simulink model "pattern3x3_training_2023clock"  (R2024a)
settings: Solver=FixedStepAuto  StartTime=0.0  StopTime=2  FixedStep=0.000005  RelTol=1e-3
model workspace (MAT data in the model file):
  part1_v1 = 1
values from neighbouring files (symbols this model uses):
  full_pattern = load('Pattern4_250.CSV')    [model_setup4.m]
  max_weight2 = 255    [model_setup4.m]
  min_weight2 = 150    [model_setup4.m]
  Th_minus_count2 = 10    [model_setup4.m]    (also in model_setup_test.m = 5)
  Th_plus_count2 = 20    [model_setup4.m]    (also in model_setup_test.m)
libraries: simulink x1
(part 6 of 9)

== system pattern3x3_training_2023clock/Synapse11/Clock2 ==
  clock : Inport
  "Reset " : Inport  Port=2
  Memory2 : Memory
  NOT1 : Logic  Operator=NOT  IconShape=distinctive  AllPortsSameDT=off  OutDataTypeStr=boolean
  Product1 : Product
  Triggered Subsystem1 : Subsystem  TreatAsAtomicUnit=on
  T : Outport  VectorParamsAs1DForOutWhenUnconnected=off
  wires:
  Memory2/1 -> Triggered Subsystem1/1(In1)
  Product1/1 -> T/1, Memory2/1
  "Reset "/1 -> NOT1/1
  Triggered Subsystem1/1(Out1) -> Product1/1
  NOT1/1 -> Product1/2
  clock/1 -> Triggered Subsystem1/Trigger

== system pattern3x3_training_2023clock/Synapse11/Clock3 ==
  clock : Inport
  "Reset " : Inport  Port=2
  Memory2 : Memory
  NOT1 : Logic  Operator=NOT  IconShape=distinctive  AllPortsSameDT=off  OutDataTypeStr=boolean
  Product1 : Product
  Triggered Subsystem1 : Subsystem  TreatAsAtomicUnit=on
  T : Outport  VectorParamsAs1DForOutWhenUnconnected=off
  wires:
  Memory2/1 -> Triggered Subsystem1/1(In1)
  Product1/1 -> T/1, Memory2/1
  "Reset "/1 -> NOT1/1
  Triggered Subsystem1/1(Out1) -> Product1/1
  NOT1/1 -> Product1/2
  clock/1 -> Triggered Subsystem1/Trigger

== system pattern3x3_training_2023clock/Synapse11/Subsystem ==
  delta_weight : Inport
  before_weight : Inport  Port=2
  Trigger : TriggerPort  VariantControl=(inherit)  PortDimensions=1
  Sum : Sum  Inputs=|++
  weight : Outport
  wires:
  delta_weight/1 -> Sum/1
  Sum/1 -> weight/1
  before_weight/1 -> Sum/2

== system pattern3x3_training_2023clock/Synapse12/Clock1 ==
  clock : Inport
  "Reset " : Inport  Port=2
  Memory2 : Memory
  NOT1 : Logic  Operator=NOT  IconShape=distinctive  AllPortsSameDT=off  OutDataTypeStr=boolean
  Product1 : Product
  Triggered Subsystem1 : Subsystem  TreatAsAtomicUnit=on
  T : Outport  VectorParamsAs1DForOutWhenUnconnected=off
  wires:
  Memory2/1 -> Triggered Subsystem1/1(In1)
  Product1/1 -> T/1, Memory2/1
  "Reset "/1 -> NOT1/1
  Triggered Subsystem1/1(Out1) -> Product1/1
  NOT1/1 -> Product1/2
  clock/1 -> Triggered Subsystem1/Trigger

== system pattern3x3_training_2023clock/Synapse12/Clock2 ==
  clock : Inport
  "Reset " : Inport  Port=2
  Memory2 : Memory
  NOT1 : Logic  Operator=NOT  IconShape=distinctive  AllPortsSameDT=off  OutDataTypeStr=boolean
  Product1 : Product
  Triggered Subsystem1 : Subsystem  TreatAsAtomicUnit=on
  T : Outport  VectorParamsAs1DForOutWhenUnconnected=off
  wires:
  Memory2/1 -> Triggered Subsystem1/1(In1)
  Product1/1 -> T/1, Memory2/1
  "Reset "/1 -> NOT1/1
  Triggered Subsystem1/1(Out1) -> Product1/1
  NOT1/1 -> Product1/2
  clock/1 -> Triggered Subsystem1/Trigger

== system pattern3x3_training_2023clock/Synapse12/Clock3 ==
  clock : Inport
  "Reset " : Inport  Port=2
  Memory2 : Memory
  NOT1 : Logic  Operator=NOT  IconShape=distinctive  AllPortsSameDT=off  OutDataTypeStr=boolean
  Product1 : Product
  Triggered Subsystem1 : Subsystem  TreatAsAtomicUnit=on
  T : Outport  VectorParamsAs1DForOutWhenUnconnected=off
  wires:
  Memory2/1 -> Triggered Subsystem1/1(In1)
  Product1/1 -> T/1, Memory2/1
  "Reset "/1 -> NOT1/1
  Triggered Subsystem1/1(Out1) -> Product1/1
  NOT1/1 -> Product1/2
  clock/1 -> Triggered Subsystem1/Trigger

== system pattern3x3_training_2023clock/Synapse12/Subsystem ==
  delta_weight : Inport
  before_weight : Inport  Port=2
  Trigger : TriggerPort  VariantControl=(inherit)  PortDimensions=1
  Sum : Sum  Inputs=|++
  weight : Outport
  wires:
  delta_weight/1 -> Sum/1
  Sum/1 -> weight/1
  before_weight/1 -> Sum/2

== system pattern3x3_training_2023clock/Synapse13/Clock1 ==
  clock : Inport
  "Reset " : Inport  Port=2
  Memory2 : Memory
  NOT1 : Logic  Operator=NOT  IconShape=distinctive  AllPortsSameDT=off  OutDataTypeStr=boolean
  Product1 : Product
  Triggered Subsystem1 : Subsystem  TreatAsAtomicUnit=on
  T : Outport  VectorParamsAs1DForOutWhenUnconnected=off
  wires:
  Memory2/1 -> Triggered Subsystem1/1(In1)
  Product1/1 -> T/1, Memory2/1
  "Reset "/1 -> NOT1/1
  Triggered Subsystem1/1(Out1) -> Product1/1
  NOT1/1 -> Product1/2
  clock/1 -> Triggered Subsystem1/Trigger

== system pattern3x3_training_2023clock/Synapse13/Clock2 ==
  clock : Inport
  "Reset " : Inport  Port=2
  Memory2 : Memory
  NOT1 : Logic  Operator=NOT  IconShape=distinctive  AllPortsSameDT=off  OutDataTypeStr=boolean
  Product1 : Product
  Triggered Subsystem1 : Subsystem  TreatAsAtomicUnit=on
  T : Outport  VectorParamsAs1DForOutWhenUnconnected=off
  wires:
  Memory2/1 -> Triggered Subsystem1/1(In1)
  Product1/1 -> T/1, Memory2/1
  "Reset "/1 -> NOT1/1
  Triggered Subsystem1/1(Out1) -> Product1/1
  NOT1/1 -> Product1/2
  clock/1 -> Triggered Subsystem1/Trigger

== system pattern3x3_training_2023clock/Synapse13/Clock3 ==
  clock : Inport
  "Reset " : Inport  Port=2
  Memory2 : Memory
  NOT1 : Logic  Operator=NOT  IconShape=distinctive  AllPortsSameDT=off  OutDataTypeStr=boolean
  Product1 : Product
  Triggered Subsystem1 : Subsystem  TreatAsAtomicUnit=on
  T : Outport  VectorParamsAs1DForOutWhenUnconnected=off
  wires:
  Memory2/1 -> Triggered Subsystem1/1(In1)
  Product1/1 -> T/1, Memory2/1
  "Reset "/1 -> NOT1/1
  Triggered Subsystem1/1(Out1) -> Product1/1
  NOT1/1 -> Product1/2
  clock/1 -> Triggered Subsystem1/Trigger

== system pattern3x3_training_2023clock/Synapse13/Subsystem ==
  delta_weight : Inport
  before_weight : Inport  Port=2
  Trigger : TriggerPort  VariantControl=(inherit)  PortDimensions=1
  Sum : Sum  Inputs=|++
  weight : Outport
  wires:
  delta_weight/1 -> Sum/1
  Sum/1 -> weight/1
  before_weight/1 -> Sum/2

== system pattern3x3_training_2023clock/Synapse14/Clock1 ==
  clock : Inport
  "Reset " : Inport  Port=2
  Memory2 : Memory
  NOT1 : Logic  Operator=NOT  IconShape=distinctive  AllPortsSameDT=off  OutDataTypeStr=boolean
  Product1 : Product
  Triggered Subsystem1 : Subsystem  TreatAsAtomicUnit=on
  T : Outport  VectorParamsAs1DForOutWhenUnconnected=off
  wires:
  Memory2/1 -> Triggered Subsystem1/1(In1)
  Product1/1 -> T/1, Memory2/1
  "Reset "/1 -> NOT1/1
  Triggered Subsystem1/1(Out1) -> Product1/1
  NOT1/1 -> Product1/2
  clock/1 -> Triggered Subsystem1/Trigger

== system pattern3x3_training_2023clock/Synapse14/Clock2 ==
  clock : Inport
  "Reset " : Inport  Port=2
  Memory2 : Memory
  NOT1 : Logic  Operator=NOT  IconShape=distinctive  AllPortsSameDT=off  OutDataTypeStr=boolean
  Product1 : Product
  Triggered Subsystem1 : Subsystem  TreatAsAtomicUnit=on
  T : Outport  VectorParamsAs1DForOutWhenUnconnected=off
  wires:
  Memory2/1 -> Triggered Subsystem1/1(In1)
  Product1/1 -> T/1, Memory2/1
  "Reset "/1 -> NOT1/1
  Triggered Subsystem1/1(Out1) -> Product1/1
  NOT1/1 -> Product1/2
  clock/1 -> Triggered Subsystem1/Trigger

== system pattern3x3_training_2023clock/Synapse14/Clock3 ==
  clock : Inport
  "Reset " : Inport  Port=2
  Memory2 : Memory
  NOT1 : Logic  Operator=NOT  IconShape=distinctive  AllPortsSameDT=off  OutDataTypeStr=boolean
  Product1 : Product
  Triggered Subsystem1 : Subsystem  TreatAsAtomicUnit=on
  T : Outport  VectorParamsAs1DForOutWhenUnconnected=off
  wires:
  Memory2/1 -> Triggered Subsystem1/1(In1)
  Product1/1 -> T/1, Memory2/1
  "Reset "/1 -> NOT1/1
  Triggered Subsystem1/1(Out1) -> Product1/1
  NOT1/1 -> Product1/2
  clock/1 -> Triggered Subsystem1/Trigger

== system pattern3x3_training_2023clock/Synapse14/Subsystem ==
  delta_weight : Inport
  before_weight : Inport  Port=2
  Trigger : TriggerPort  VariantControl=(inherit)  PortDimensions=1
  Sum : Sum  Inputs=|++
  weight : Outport
  wires:
  delta_weight/1 -> Sum/1
  Sum/1 -> weight/1
  before_weight/1 -> Sum/2

== system pattern3x3_training_2023clock/Synapse15/Clock1 ==
  clock : Inport
  "Reset " : Inport  Port=2
  Memory2 : Memory
  NOT1 : Logic  Operator=NOT  IconShape=distinctive  AllPortsSameDT=off  OutDataTypeStr=boolean
  Product1 : Product
  Triggered Subsystem1 : Subsystem  TreatAsAtomicUnit=on
  T : Outport  VectorParamsAs1DForOutWhenUnconnected=off
  wires:
  Memory2/1 -> Triggered Subsystem1/1(In1)
  Product1/1 -> T/1, Memory2/1
  "Reset "/1 -> NOT1/1
  Triggered Subsystem1/1(Out1) -> Product1/1
  NOT1/1 -> Product1/2
  clock/1 -> Triggered Subsystem1/Trigger

== system pattern3x3_training_2023clock/Synapse15/Clock2 ==
  clock : Inport
  "Reset " : Inport  Port=2
  Memory2 : Memory
  NOT1 : Logic  Operator=NOT  IconShape=distinctive  AllPortsSameDT=off  OutDataTypeStr=boolean
  Product1 : Product
  Triggered Subsystem1 : Subsystem  TreatAsAtomicUnit=on
  T : Outport  VectorParamsAs1DForOutWhenUnconnected=off
  wires:
  Memory2/1 -> Triggered Subsystem1/1(In1)
  Product1/1 -> T/1, Memory2/1
  "Reset "/1 -> NOT1/1
  Triggered Subsystem1/1(Out1) -> Product1/1
  NOT1/1 -> Product1/2
  clock/1 -> Triggered Subsystem1/Trigger

== system pattern3x3_training_2023clock/Synapse15/Clock3 ==
  clock : Inport
  "Reset " : Inport  Port=2
  Memory2 : Memory
  NOT1 : Logic  Operator=NOT  IconShape=distinctive  AllPortsSameDT=off  OutDataTypeStr=boolean
  Product1 : Product
  Triggered Subsystem1 : Subsystem  TreatAsAtomicUnit=on
  T : Outport  VectorParamsAs1DForOutWhenUnconnected=off
  wires:
  Memory2/1 -> Triggered Subsystem1/1(In1)
  Product1/1 -> T/1, Memory2/1
  "Reset "/1 -> NOT1/1
  Triggered Subsystem1/1(Out1) -> Product1/1
  NOT1/1 -> Product1/2
  clock/1 -> Triggered Subsystem1/Trigger

== system pattern3x3_training_2023clock/Synapse15/Subsystem ==
  delta_weight : Inport
  before_weight : Inport  Port=2
  Trigger : TriggerPort  VariantControl=(inherit)  PortDimensions=1
  Sum : Sum  Inputs=|++
  weight : Outport
  wires:
  delta_weight/1 -> Sum/1
  Sum/1 -> weight/1
  before_weight/1 -> Sum/2

== system pattern3x3_training_2023clock/Synapse16/Clock1 ==
  clock : Inport
  "Reset " : Inport  Port=2
  Memory2 : Memory
  NOT1 : Logic  Operator=NOT  IconShape=distinctive  AllPortsSameDT=off  OutDataTypeStr=boolean
  Product1 : Product
  Triggered Subsystem1 : Subsystem  TreatAsAtomicUnit=on
  T : Outport  VectorParamsAs1DForOutWhenUnconnected=off
  wires:
  Memory2/1 -> Triggered Subsystem1/1(In1)
  Product1/1 -> T/1, Memory2/1
  "Reset "/1 -> NOT1/1
  Triggered Subsystem1/1(Out1) -> Product1/1
  NOT1/1 -> Product1/2
  clock/1 -> Triggered Subsystem1/Trigger

== system pattern3x3_training_2023clock/Synapse16/Clock2 ==
  clock : Inport
  "Reset " : Inport  Port=2
  Memory2 : Memory
  NOT1 : Logic  Operator=NOT  IconShape=distinctive  AllPortsSameDT=off  OutDataTypeStr=boolean
  Product1 : Product
  Triggered Subsystem1 : Subsystem  TreatAsAtomicUnit=on
  T : Outport  VectorParamsAs1DForOutWhenUnconnected=off
  wires:
  Memory2/1 -> Triggered Subsystem1/1(In1)
  Product1/1 -> T/1, Memory2/1
  "Reset "/1 -> NOT1/1
  Triggered Subsystem1/1(Out1) -> Product1/1
  NOT1/1 -> Product1/2
  clock/1 -> Triggered Subsystem1/Trigger

== system pattern3x3_training_2023clock/Synapse16/Clock3 ==
  clock : Inport
  "Reset " : Inport  Port=2
  Memory2 : Memory
  NOT1 : Logic  Operator=NOT  IconShape=distinctive  AllPortsSameDT=off  OutDataTypeStr=boolean
  Product1 : Product
  Triggered Subsystem1 : Subsystem  TreatAsAtomicUnit=on
  T : Outport  VectorParamsAs1DForOutWhenUnconnected=off
  wires:
  Memory2/1 -> Triggered Subsystem1/1(In1)
  Product1/1 -> T/1, Memory2/1
  "Reset "/1 -> NOT1/1
  Triggered Subsystem1/1(Out1) -> Product1/1
  NOT1/1 -> Product1/2
  clock/1 -> Triggered Subsystem1/Trigger

== system pattern3x3_training_2023clock/Synapse16/Subsystem ==
  delta_weight : Inport
  before_weight : Inport  Port=2
  Trigger : TriggerPort  VariantControl=(inherit)  PortDimensions=1
  Sum : Sum  Inputs=|++
  weight : Outport
  wires:
  delta_weight/1 -> Sum/1
  Sum/1 -> weight/1
  before_weight/1 -> Sum/2

== system pattern3x3_training_2023clock/Synapse17/Clock1 ==
  clock : Inport
  "Reset " : Inport  Port=2
  Memory2 : Memory
  NOT1 : Logic  Operator=NOT  IconShape=distinctive  AllPortsSameDT=off  OutDataTypeStr=boolean
  Product1 : Product
  Triggered Subsystem1 : Subsystem  TreatAsAtomicUnit=on
  T : Outport  VectorParamsAs1DForOutWhenUnconnected=off
  wires:
  Memory2/1 -> Triggered Subsystem1/1(In1)
  Product1/1 -> T/1, Memory2/1
  "Reset "/1 -> NOT1/1
  Triggered Subsystem1/1(Out1) -> Product1/1
  NOT1/1 -> Product1/2
  clock/1 -> Triggered Subsystem1/Trigger

== system pattern3x3_training_2023clock/Synapse17/Clock2 ==
  clock : Inport
  "Reset " : Inport  Port=2
  Memory2 : Memory
  NOT1 : Logic  Operator=NOT  IconShape=distinctive  AllPortsSameDT=off  OutDataTypeStr=boolean
  Product1 : Product
  Triggered Subsystem1 : Subsystem  TreatAsAtomicUnit=on
  T : Outport  VectorParamsAs1DForOutWhenUnconnected=off
  wires:
  Memory2/1 -> Triggered Subsystem1/1(In1)
  Product1/1 -> T/1, Memory2/1
  "Reset "/1 -> NOT1/1
  Triggered Subsystem1/1(Out1) -> Product1/1
  NOT1/1 -> Product1/2
  clock/1 -> Triggered Subsystem1/Trigger

== system pattern3x3_training_2023clock/Synapse17/Clock3 ==
  clock : Inport
  "Reset " : Inport  Port=2
  Memory2 : Memory
  NOT1 : Logic  Operator=NOT  IconShape=distinctive  AllPortsSameDT=off  OutDataTypeStr=boolean
  Product1 : Product
  Triggered Subsystem1 : Subsystem  TreatAsAtomicUnit=on
  T : Outport  VectorParamsAs1DForOutWhenUnconnected=off
  wires:
  Memory2/1 -> Triggered Subsystem1/1(In1)
  Product1/1 -> T/1, Memory2/1
  "Reset "/1 -> NOT1/1
  Triggered Subsystem1/1(Out1) -> Product1/1
  NOT1/1 -> Product1/2
  clock/1 -> Triggered Subsystem1/Trigger

== system pattern3x3_training_2023clock/Synapse17/Subsystem ==
  delta_weight : Inport
  before_weight : Inport  Port=2
  Trigger : TriggerPort  VariantControl=(inherit)  PortDimensions=1
  Sum : Sum  Inputs=|++
  weight : Outport
  wires:
  delta_weight/1 -> Sum/1
  Sum/1 -> weight/1
  before_weight/1 -> Sum/2

== system pattern3x3_training_2023clock/Synapse18/Clock1 ==
  clock : Inport
  "Reset " : Inport  Port=2
  Memory2 : Memory
  NOT1 : Logic  Operator=NOT  IconShape=distinctive  AllPortsSameDT=off  OutDataTypeStr=boolean
  Product1 : Product
  Triggered Subsystem1 : Subsystem  TreatAsAtomicUnit=on
  T : Outport  VectorParamsAs1DForOutWhenUnconnected=off
  wires:
  Memory2/1 -> Triggered Subsystem1/1(In1)
  Product1/1 -> T/1, Memory2/1
  "Reset "/1 -> NOT1/1
  Triggered Subsystem1/1(Out1) -> Product1/1
  NOT1/1 -> Product1/2
  clock/1 -> Triggered Subsystem1/Trigger

== system pattern3x3_training_2023clock/Synapse18/Clock2 ==
  clock : Inport
  "Reset " : Inport  Port=2
  Memory2 : Memory
  NOT1 : Logic  Operator=NOT  IconShape=distinctive  AllPortsSameDT=off  OutDataTypeStr=boolean
  Product1 : Product
  Triggered Subsystem1 : Subsystem  TreatAsAtomicUnit=on
  T : Outport  VectorParamsAs1DForOutWhenUnconnected=off
  wires:
  Memory2/1 -> Triggered Subsystem1/1(In1)
  Product1/1 -> T/1, Memory2/1
  "Reset "/1 -> NOT1/1
  Triggered Subsystem1/1(Out1) -> Product1/1
  NOT1/1 -> Product1/2
  clock/1 -> Triggered Subsystem1/Trigger

== system pattern3x3_training_2023clock/Synapse18/Clock3 ==
  clock : Inport
  "Reset " : Inport  Port=2
  Memory2 : Memory
  NOT1 : Logic  Operator=NOT  IconShape=distinctive  AllPortsSameDT=off  OutDataTypeStr=boolean
  Product1 : Product
  Triggered Subsystem1 : Subsystem  TreatAsAtomicUnit=on
  T : Outport  VectorParamsAs1DForOutWhenUnconnected=off
  wires:
  Memory2/1 -> Triggered Subsystem1/1(In1)
  Product1/1 -> T/1, Memory2/1
  "Reset "/1 -> NOT1/1
  Triggered Subsystem1/1(Out1) -> Product1/1
  NOT1/1 -> Product1/2
  clock/1 -> Triggered Subsystem1/Trigger

== system pattern3x3_training_2023clock/Synapse18/Subsystem ==
  delta_weight : Inport
  before_weight : Inport  Port=2
  Trigger : TriggerPort  VariantControl=(inherit)  PortDimensions=1
  Sum : Sum  Inputs=|++
  weight : Outport
  wires:
  delta_weight/1 -> Sum/1
  Sum/1 -> weight/1
  before_weight/1 -> Sum/2

== system pattern3x3_training_2023clock/Synapse19/Clock1 ==
  clock : Inport
  "Reset " : Inport  Port=2
  Memory2 : Memory
  NOT1 : Logic  Operator=NOT  IconShape=distinctive  AllPortsSameDT=off  OutDataTypeStr=boolean
  Product1 : Product
  Triggered Subsystem1 : Subsystem  TreatAsAtomicUnit=on
  T : Outport  VectorParamsAs1DForOutWhenUnconnected=off
  wires:
  Memory2/1 -> Triggered Subsystem1/1(In1)
  Product1/1 -> T/1, Memory2/1
  "Reset "/1 -> NOT1/1
  Triggered Subsystem1/1(Out1) -> Product1/1
  NOT1/1 -> Product1/2
  clock/1 -> Triggered Subsystem1/Trigger

== system pattern3x3_training_2023clock/Synapse19/Clock2 ==
  clock : Inport
  "Reset " : Inport  Port=2
  Memory2 : Memory
  NOT1 : Logic  Operator=NOT  IconShape=distinctive  AllPortsSameDT=off  OutDataTypeStr=boolean
  Product1 : Product
  Triggered Subsystem1 : Subsystem  TreatAsAtomicUnit=on
  T : Outport  VectorParamsAs1DForOutWhenUnconnected=off
  wires:
  Memory2/1 -> Triggered Subsystem1/1(In1)
  Product1/1 -> T/1, Memory2/1
  "Reset "/1 -> NOT1/1
  Triggered Subsystem1/1(Out1) -> Product1/1
  NOT1/1 -> Product1/2
  clock/1 -> Triggered Subsystem1/Trigger

== system pattern3x3_training_2023clock/Synapse19/Clock3 ==
  clock : Inport
  "Reset " : Inport  Port=2
  Memory2 : Memory
  NOT1 : Logic  Operator=NOT  IconShape=distinctive  AllPortsSameDT=off  OutDataTypeStr=boolean
  Product1 : Product
  Triggered Subsystem1 : Subsystem  TreatAsAtomicUnit=on
  T : Outport  VectorParamsAs1DForOutWhenUnconnected=off
  wires:
  Memory2/1 -> Triggered Subsystem1/1(In1)
  Product1/1 -> T/1, Memory2/1
  "Reset "/1 -> NOT1/1
  Triggered Subsystem1/1(Out1) -> Product1/1
  NOT1/1 -> Product1/2
  clock/1 -> Triggered Subsystem1/Trigger

== system pattern3x3_training_2023clock/Synapse19/Subsystem ==
  delta_weight : Inport
  before_weight : Inport  Port=2
  Trigger : TriggerPort  VariantControl=(inherit)  PortDimensions=1
  Sum : Sum  Inputs=|++
  weight : Outport
  wires:
  delta_weight/1 -> Sum/1
  Sum/1 -> weight/1
  before_weight/1 -> Sum/2

== system pattern3x3_training_2023clock/Synapse2/Clock1 ==
  clock : Inport
  "Reset " : Inport  Port=2
  Memory2 : Memory
  NOT1 : Logic  Operator=NOT  IconShape=distinctive  AllPortsSameDT=off  OutDataTypeStr=boolean
  Product1 : Product
  Triggered Subsystem1 : Subsystem  TreatAsAtomicUnit=on
  T : Outport  VectorParamsAs1DForOutWhenUnconnected=off
  wires:
  Memory2/1 -> Triggered Subsystem1/1(In1)
  Product1/1 -> T/1, Memory2/1
  "Reset "/1 -> NOT1/1
  Triggered Subsystem1/1(Out1) -> Product1/1
  NOT1/1 -> Product1/2
  clock/1 -> Triggered Subsystem1/Trigger

== system pattern3x3_training_2023clock/Synapse2/Clock2 ==
  clock : Inport
  "Reset " : Inport  Port=2
  Memory2 : Memory
  NOT1 : Logic  Operator=NOT  IconShape=distinctive  AllPortsSameDT=off  OutDataTypeStr=boolean
  Product1 : Product
  Triggered Subsystem1 : Subsystem  TreatAsAtomicUnit=on
  T : Outport  VectorParamsAs1DForOutWhenUnconnected=off
  wires:
  Memory2/1 -> Triggered Subsystem1/1(In1)
  Product1/1 -> T/1, Memory2/1
  "Reset "/1 -> NOT1/1
  Triggered Subsystem1/1(Out1) -> Product1/1
  NOT1/1 -> Product1/2
  clock/1 -> Triggered Subsystem1/Trigger

== system pattern3x3_training_2023clock/Synapse2/Clock3 ==
  clock : Inport
  "Reset " : Inport  Port=2
  Memory2 : Memory
  NOT1 : Logic  Operator=NOT  IconShape=distinctive  AllPortsSameDT=off  OutDataTypeStr=boolean
  Product1 : Product
  Triggered Subsystem1 : Subsystem  TreatAsAtomicUnit=on
  T : Outport  VectorParamsAs1DForOutWhenUnconnected=off
  wires:
  Memory2/1 -> Triggered Subsystem1/1(In1)
  Product1/1 -> T/1, Memory2/1
  "Reset "/1 -> NOT1/1
  Triggered Subsystem1/1(Out1) -> Product1/1
  NOT1/1 -> Product1/2
  clock/1 -> Triggered Subsystem1/Trigger

== system pattern3x3_training_2023clock/Synapse2/Subsystem ==
  delta_weight : Inport
  before_weight : Inport  Port=2
  Trigger : TriggerPort  VariantControl=(inherit)  PortDimensions=1
  Sum : Sum  Inputs=|++
  weight : Outport
  wires:
  delta_weight/1 -> Sum/1
  Sum/1 -> weight/1
  before_weight/1 -> Sum/2

== system pattern3x3_training_2023clock/Synapse20/Clock1 ==
  clock : Inport
  "Reset " : Inport  Port=2
  Memory2 : Memory
  NOT1 : Logic  Operator=NOT  IconShape=distinctive  AllPortsSameDT=off  OutDataTypeStr=boolean
  Product1 : Product
  Triggered Subsystem1 : Subsystem  TreatAsAtomicUnit=on
  T : Outport  VectorParamsAs1DForOutWhenUnconnected=off
  wires:
  Memory2/1 -> Triggered Subsystem1/1(In1)
  Product1/1 -> T/1, Memory2/1
  "Reset "/1 -> NOT1/1
  Triggered Subsystem1/1(Out1) -> Product1/1
  NOT1/1 -> Product1/2
  clock/1 -> Triggered Subsystem1/Trigger

== system pattern3x3_training_2023clock/Synapse20/Clock2 ==
  clock : Inport
  "Reset " : Inport  Port=2
  Memory2 : Memory
  NOT1 : Logic  Operator=NOT  IconShape=distinctive  AllPortsSameDT=off  OutDataTypeStr=boolean
  Product1 : Product
  Triggered Subsystem1 : Subsystem  TreatAsAtomicUnit=on
  T : Outport  VectorParamsAs1DForOutWhenUnconnected=off
  wires:
  Memory2/1 -> Triggered Subsystem1/1(In1)
  Product1/1 -> T/1, Memory2/1
  "Reset "/1 -> NOT1/1
  Triggered Subsystem1/1(Out1) -> Product1/1
  NOT1/1 -> Product1/2
  clock/1 -> Triggered Subsystem1/Trigger

== system pattern3x3_training_2023clock/Synapse20/Clock3 ==
  clock : Inport
  "Reset " : Inport  Port=2
  Memory2 : Memory
  NOT1 : Logic  Operator=NOT  IconShape=distinctive  AllPortsSameDT=off  OutDataTypeStr=boolean
  Product1 : Product
  Triggered Subsystem1 : Subsystem  TreatAsAtomicUnit=on
  T : Outport  VectorParamsAs1DForOutWhenUnconnected=off
  wires:
  Memory2/1 -> Triggered Subsystem1/1(In1)
  Product1/1 -> T/1, Memory2/1
  "Reset "/1 -> NOT1/1
  Triggered Subsystem1/1(Out1) -> Product1/1
  NOT1/1 -> Product1/2
  clock/1 -> Triggered Subsystem1/Trigger

== system pattern3x3_training_2023clock/Synapse20/Subsystem ==
  delta_weight : Inport
  before_weight : Inport  Port=2
  Trigger : TriggerPort  VariantControl=(inherit)  PortDimensions=1
  Sum : Sum  Inputs=|++
  weight : Outport
  wires:
  delta_weight/1 -> Sum/1
  Sum/1 -> weight/1
  before_weight/1 -> Sum/2

== system pattern3x3_training_2023clock/Synapse21/Clock1 ==
  clock : Inport
  "Reset " : Inport  Port=2
  Memory2 : Memory
  NOT1 : Logic  Operator=NOT  IconShape=distinctive  AllPortsSameDT=off  OutDataTypeStr=boolean
  Product1 : Product
  Triggered Subsystem1 : Subsystem  TreatAsAtomicUnit=on
  T : Outport  VectorParamsAs1DForOutWhenUnconnected=off
  wires:
  Memory2/1 -> Triggered Subsystem1/1(In1)
  Product1/1 -> T/1, Memory2/1
  "Reset "/1 -> NOT1/1
  Triggered Subsystem1/1(Out1) -> Product1/1
  NOT1/1 -> Product1/2
  clock/1 -> Triggered Subsystem1/Trigger

== system pattern3x3_training_2023clock/Synapse21/Clock2 ==
  clock : Inport
  "Reset " : Inport  Port=2
  Memory2 : Memory
  NOT1 : Logic  Operator=NOT  IconShape=distinctive  AllPortsSameDT=off  OutDataTypeStr=boolean
  Product1 : Product
  Triggered Subsystem1 : Subsystem  TreatAsAtomicUnit=on
  T : Outport  VectorParamsAs1DForOutWhenUnconnected=off
  wires:
  Memory2/1 -> Triggered Subsystem1/1(In1)
  Product1/1 -> T/1, Memory2/1
  "Reset "/1 -> NOT1/1
  Triggered Subsystem1/1(Out1) -> Product1/1
  NOT1/1 -> Product1/2
  clock/1 -> Triggered Subsystem1/Trigger

== system pattern3x3_training_2023clock/Synapse21/Clock3 ==
  clock : Inport
  "Reset " : Inport  Port=2
  Memory2 : Memory
  NOT1 : Logic  Operator=NOT  IconShape=distinctive  AllPortsSameDT=off  OutDataTypeStr=boolean
  Product1 : Product
  Triggered Subsystem1 : Subsystem  TreatAsAtomicUnit=on
  T : Outport  VectorParamsAs1DForOutWhenUnconnected=off
  wires:
  Memory2/1 -> Triggered Subsystem1/1(In1)
  Product1/1 -> T/1, Memory2/1
  "Reset "/1 -> NOT1/1
  Triggered Subsystem1/1(Out1) -> Product1/1
  NOT1/1 -> Product1/2
  clock/1 -> Triggered Subsystem1/Trigger

== system pattern3x3_training_2023clock/Synapse21/Subsystem ==
  delta_weight : Inport
  before_weight : Inport  Port=2
  Trigger : TriggerPort  VariantControl=(inherit)  PortDimensions=1
  Sum : Sum  Inputs=|++
  weight : Outport
  wires:
  delta_weight/1 -> Sum/1
  Sum/1 -> weight/1
  before_weight/1 -> Sum/2

== system pattern3x3_training_2023clock/Synapse22/Clock1 ==
  clock : Inport
  "Reset " : Inport  Port=2
  Memory2 : Memory
  NOT1 : Logic  Operator=NOT  IconShape=distinctive  AllPortsSameDT=off  OutDataTypeStr=boolean
  Product1 : Product
  Triggered Subsystem1 : Subsystem  TreatAsAtomicUnit=on
  T : Outport  VectorParamsAs1DForOutWhenUnconnected=off
  wires:
  Memory2/1 -> Triggered Subsystem1/1(In1)
  Product1/1 -> T/1, Memory2/1
  "Reset "/1 -> NOT1/1
  Triggered Subsystem1/1(Out1) -> Product1/1
  NOT1/1 -> Product1/2
  clock/1 -> Triggered Subsystem1/Trigger

== system pattern3x3_training_2023clock/Synapse22/Clock2 ==
  clock : Inport
  "Reset " : Inport  Port=2
  Memory2 : Memory
  NOT1 : Logic  Operator=NOT  IconShape=distinctive  AllPortsSameDT=off  OutDataTypeStr=boolean
  Product1 : Product
  Triggered Subsystem1 : Subsystem  TreatAsAtomicUnit=on
  T : Outport  VectorParamsAs1DForOutWhenUnconnected=off
  wires:
  Memory2/1 -> Triggered Subsystem1/1(In1)
  Product1/1 -> T/1, Memory2/1
  "Reset "/1 -> NOT1/1
  Triggered Subsystem1/1(Out1) -> Product1/1
  NOT1/1 -> Product1/2
  clock/1 -> Triggered Subsystem1/Trigger

== system pattern3x3_training_2023clock/Synapse22/Clock3 ==
  clock : Inport
  "Reset " : Inport  Port=2
  Memory2 : Memory
  NOT1 : Logic  Operator=NOT  IconShape=distinctive  AllPortsSameDT=off  OutDataTypeStr=boolean
  Product1 : Product
  Triggered Subsystem1 : Subsystem  TreatAsAtomicUnit=on
  T : Outport  VectorParamsAs1DForOutWhenUnconnected=off
  wires:
  Memory2/1 -> Triggered Subsystem1/1(In1)
  Product1/1 -> T/1, Memory2/1
  "Reset "/1 -> NOT1/1
  Triggered Subsystem1/1(Out1) -> Product1/1
  NOT1/1 -> Product1/2
  clock/1 -> Triggered Subsystem1/Trigger

== system pattern3x3_training_2023clock/Synapse22/Subsystem ==
  delta_weight : Inport
  before_weight : Inport  Port=2
  Trigger : TriggerPort  VariantControl=(inherit)  PortDimensions=1
  Sum : Sum  Inputs=|++
  weight : Outport
  wires:
  delta_weight/1 -> Sum/1
  Sum/1 -> weight/1
  before_weight/1 -> Sum/2

== system pattern3x3_training_2023clock/Synapse23/Clock1 ==
  clock : Inport
  "Reset " : Inport  Port=2
  Memory2 : Memory
  NOT1 : Logic  Operator=NOT  IconShape=distinctive  AllPortsSameDT=off  OutDataTypeStr=boolean
  Product1 : Product
  Triggered Subsystem1 : Subsystem  TreatAsAtomicUnit=on
  T : Outport  VectorParamsAs1DForOutWhenUnconnected=off
  wires:
  Memory2/1 -> Triggered Subsystem1/1(In1)
  Product1/1 -> T/1, Memory2/1
  "Reset "/1 -> NOT1/1
  Triggered Subsystem1/1(Out1) -> Product1/1
  NOT1/1 -> Product1/2
  clock/1 -> Triggered Subsystem1/Trigger

== system pattern3x3_training_2023clock/Synapse23/Clock2 ==
  clock : Inport
  "Reset " : Inport  Port=2
  Memory2 : Memory
  NOT1 : Logic  Operator=NOT  IconShape=distinctive  AllPortsSameDT=off  OutDataTypeStr=boolean
  Product1 : Product
  Triggered Subsystem1 : Subsystem  TreatAsAtomicUnit=on
  T : Outport  VectorParamsAs1DForOutWhenUnconnected=off
  wires:
  Memory2/1 -> Triggered Subsystem1/1(In1)
  Product1/1 -> T/1, Memory2/1
  "Reset "/1 -> NOT1/1
  Triggered Subsystem1/1(Out1) -> Product1/1
  NOT1/1 -> Product1/2
  clock/1 -> Triggered Subsystem1/Trigger

== system pattern3x3_training_2023clock/Synapse23/Clock3 ==
  clock : Inport
  "Reset " : Inport  Port=2
  Memory2 : Memory
  NOT1 : Logic  Operator=NOT  IconShape=distinctive  AllPortsSameDT=off  OutDataTypeStr=boolean
  Product1 : Product
  Triggered Subsystem1 : Subsystem  TreatAsAtomicUnit=on
  T : Outport  VectorParamsAs1DForOutWhenUnconnected=off
  wires:
  Memory2/1 -> Triggered Subsystem1/1(In1)
  Product1/1 -> T/1, Memory2/1
  "Reset "/1 -> NOT1/1
  Triggered Subsystem1/1(Out1) -> Product1/1
  NOT1/1 -> Product1/2
  clock/1 -> Triggered Subsystem1/Trigger

== system pattern3x3_training_2023clock/Synapse23/Subsystem ==
  delta_weight : Inport
  before_weight : Inport  Port=2
  Trigger : TriggerPort  VariantControl=(inherit)  PortDimensions=1
  Sum : Sum  Inputs=|++
  weight : Outport
  wires:
  delta_weight/1 -> Sum/1
  Sum/1 -> weight/1
  before_weight/1 -> Sum/2

== system pattern3x3_training_2023clock/Synapse24/Clock1 ==
  clock : Inport
  "Reset " : Inport  Port=2
  Memory2 : Memory
  NOT1 : Logic  Operator=NOT  IconShape=distinctive  AllPortsSameDT=off  OutDataTypeStr=boolean
  Product1 : Product
  Triggered Subsystem1 : Subsystem  TreatAsAtomicUnit=on
  T : Outport  VectorParamsAs1DForOutWhenUnconnected=off
  wires:
  Memory2/1 -> Triggered Subsystem1/1(In1)
  Product1/1 -> T/1, Memory2/1
  "Reset "/1 -> NOT1/1
  Triggered Subsystem1/1(Out1) -> Product1/1
  NOT1/1 -> Product1/2
  clock/1 -> Triggered Subsystem1/Trigger

== system pattern3x3_training_2023clock/Synapse24/Clock2 ==
  clock : Inport
  "Reset " : Inport  Port=2
  Memory2 : Memory
  NOT1 : Logic  Operator=NOT  IconShape=distinctive  AllPortsSameDT=off  OutDataTypeStr=boolean
  Product1 : Product
  Triggered Subsystem1 : Subsystem  TreatAsAtomicUnit=on
  T : Outport  VectorParamsAs1DForOutWhenUnconnected=off
  wires:
  Memory2/1 -> Triggered Subsystem1/1(In1)
  Product1/1 -> T/1, Memory2/1
  "Reset "/1 -> NOT1/1
  Triggered Subsystem1/1(Out1) -> Product1/1
  NOT1/1 -> Product1/2
  clock/1 -> Triggered Subsystem1/Trigger

== system pattern3x3_training_2023clock/Synapse24/Clock3 ==
  clock : Inport
  "Reset " : Inport  Port=2
  Memory2 : Memory
  NOT1 : Logic  Operator=NOT  IconShape=distinctive  AllPortsSameDT=off  OutDataTypeStr=boolean
  Product1 : Product
  Triggered Subsystem1 : Subsystem  TreatAsAtomicUnit=on
  T : Outport  VectorParamsAs1DForOutWhenUnconnected=off
  wires:
  Memory2/1 -> Triggered Subsystem1/1(In1)
  Product1/1 -> T/1, Memory2/1
  "Reset "/1 -> NOT1/1
  Triggered Subsystem1/1(Out1) -> Product1/1
  NOT1/1 -> Product1/2
  clock/1 -> Triggered Subsystem1/Trigger

== system pattern3x3_training_2023clock/Synapse24/Subsystem ==
  delta_weight : Inport
  before_weight : Inport  Port=2
  Trigger : TriggerPort  VariantControl=(inherit)  PortDimensions=1
  Sum : Sum  Inputs=|++
  weight : Outport
  wires:
  delta_weight/1 -> Sum/1
  Sum/1 -> weight/1
  before_weight/1 -> Sum/2

== system pattern3x3_training_2023clock/Synapse25/Clock1 ==
  clock : Inport
  "Reset " : Inport  Port=2
  Memory2 : Memory
  NOT1 : Logic  Operator=NOT  IconShape=distinctive  AllPortsSameDT=off  OutDataTypeStr=boolean
  Product1 : Product
  Triggered Subsystem1 : Subsystem  TreatAsAtomicUnit=on
  T : Outport  VectorParamsAs1DForOutWhenUnconnected=off
  wires:
  Memory2/1 -> Triggered Subsystem1/1(In1)
  Product1/1 -> T/1, Memory2/1
  "Reset "/1 -> NOT1/1
  Triggered Subsystem1/1(Out1) -> Product1/1
  NOT1/1 -> Product1/2
  clock/1 -> Triggered Subsystem1/Trigger

== system pattern3x3_training_2023clock/Synapse25/Clock2 ==
  clock : Inport
  "Reset " : Inport  Port=2
  Memory2 : Memory
  NOT1 : Logic  Operator=NOT  IconShape=distinctive  AllPortsSameDT=off  OutDataTypeStr=boolean
  Product1 : Product
  Triggered Subsystem1 : Subsystem  TreatAsAtomicUnit=on
  T : Outport  VectorParamsAs1DForOutWhenUnconnected=off
  wires:
  Memory2/1 -> Triggered Subsystem1/1(In1)
  Product1/1 -> T/1, Memory2/1
  "Reset "/1 -> NOT1/1
  Triggered Subsystem1/1(Out1) -> Product1/1
  NOT1/1 -> Product1/2
  clock/1 -> Triggered Subsystem1/Trigger

== system pattern3x3_training_2023clock/Synapse25/Clock3 ==
  clock : Inport
  "Reset " : Inport  Port=2
  Memory2 : Memory
  NOT1 : Logic  Operator=NOT  IconShape=distinctive  AllPortsSameDT=off  OutDataTypeStr=boolean
  Product1 : Product
  Triggered Subsystem1 : Subsystem  TreatAsAtomicUnit=on
  T : Outport  VectorParamsAs1DForOutWhenUnconnected=off
  wires:
  Memory2/1 -> Triggered Subsystem1/1(In1)
  Product1/1 -> T/1, Memory2/1
  "Reset "/1 -> NOT1/1
  Triggered Subsystem1/1(Out1) -> Product1/1
  NOT1/1 -> Product1/2
  clock/1 -> Triggered Subsystem1/Trigger

== system pattern3x3_training_2023clock/Synapse25/Subsystem ==
  delta_weight : Inport
  before_weight : Inport  Port=2
  Trigger : TriggerPort  VariantControl=(inherit)  PortDimensions=1
  Sum : Sum  Inputs=|++
  weight : Outport
  wires:
  delta_weight/1 -> Sum/1
  Sum/1 -> weight/1
  before_weight/1 -> Sum/2

== system pattern3x3_training_2023clock/Synapse26/Clock1 ==
  clock : Inport
  "Reset " : Inport  Port=2
  Memory2 : Memory
  NOT1 : Logic  Operator=NOT  IconShape=distinctive  AllPortsSameDT=off  OutDataTypeStr=boolean
  Product1 : Product
  Triggered Subsystem1 : Subsystem  TreatAsAtomicUnit=on
  T : Outport  VectorParamsAs1DForOutWhenUnconnected=off
  wires:
  Memory2/1 -> Triggered Subsystem1/1(In1)
  Product1/1 -> T/1, Memory2/1
  "Reset "/1 -> NOT1/1
  Triggered Subsystem1/1(Out1) -> Product1/1
  NOT1/1 -> Product1/2
  clock/1 -> Triggered Subsystem1/Trigger

== system pattern3x3_training_2023clock/Synapse26/Clock2 ==
  clock : Inport
  "Reset " : Inport  Port=2
  Memory2 : Memory
  NOT1 : Logic  Operator=NOT  IconShape=distinctive  AllPortsSameDT=off  OutDataTypeStr=boolean
  Product1 : Product
  Triggered Subsystem1 : Subsystem  TreatAsAtomicUnit=on
  T : Outport  VectorParamsAs1DForOutWhenUnconnected=off
  wires:
  Memory2/1 -> Triggered Subsystem1/1(In1)
  Product1/1 -> T/1, Memory2/1
  "Reset "/1 -> NOT1/1
  Triggered Subsystem1/1(Out1) -> Product1/1
  NOT1/1 -> Product1/2
  clock/1 -> Triggered Subsystem1/Trigger

== system pattern3x3_training_2023clock/Synapse26/Clock3 ==
  clock : Inport
  "Reset " : Inport  Port=2
  Memory2 : Memory
  NOT1 : Logic  Operator=NOT  IconShape=distinctive  AllPortsSameDT=off  OutDataTypeStr=boolean
  Product1 : Product
  Triggered Subsystem1 : Subsystem  TreatAsAtomicUnit=on
  T : Outport  VectorParamsAs1DForOutWhenUnconnected=off
  wires:
  Memory2/1 -> Triggered Subsystem1/1(In1)
  Product1/1 -> T/1, Memory2/1
  "Reset "/1 -> NOT1/1
  Triggered Subsystem1/1(Out1) -> Product1/1
  NOT1/1 -> Product1/2
  clock/1 -> Triggered Subsystem1/Trigger

== system pattern3x3_training_2023clock/Synapse26/Subsystem ==
  delta_weight : Inport
  before_weight : Inport  Port=2
  Trigger : TriggerPort  VariantControl=(inherit)  PortDimensions=1
  Sum : Sum  Inputs=|++
  weight : Outport
  wires:
  delta_weight/1 -> Sum/1
  Sum/1 -> weight/1
  before_weight/1 -> Sum/2

== system pattern3x3_training_2023clock/Synapse27/Clock1 ==
  clock : Inport
  "Reset " : Inport  Port=2
  Memory2 : Memory
  NOT1 : Logic  Operator=NOT  IconShape=distinctive  AllPortsSameDT=off  OutDataTypeStr=boolean
  Product1 : Product
  Triggered Subsystem1 : Subsystem  TreatAsAtomicUnit=on
  T : Outport  VectorParamsAs1DForOutWhenUnconnected=off
  wires:
  Memory2/1 -> Triggered Subsystem1/1(In1)
  Product1/1 -> T/1, Memory2/1
  "Reset "/1 -> NOT1/1
  Triggered Subsystem1/1(Out1) -> Product1/1
  NOT1/1 -> Product1/2
  clock/1 -> Triggered Subsystem1/Trigger

== system pattern3x3_training_2023clock/Synapse27/Clock2 ==
  clock : Inport
  "Reset " : Inport  Port=2
  Memory2 : Memory
  NOT1 : Logic  Operator=NOT  IconShape=distinctive  AllPortsSameDT=off  OutDataTypeStr=boolean
  Product1 : Product
  Triggered Subsystem1 : Subsystem  TreatAsAtomicUnit=on
  T : Outport  VectorParamsAs1DForOutWhenUnconnected=off
  wires:
  Memory2/1 -> Triggered Subsystem1/1(In1)
  Product1/1 -> T/1, Memory2/1
  "Reset "/1 -> NOT1/1
  Triggered Subsystem1/1(Out1) -> Product1/1
  NOT1/1 -> Product1/2
  clock/1 -> Triggered Subsystem1/Trigger

== system pattern3x3_training_2023clock/Synapse27/Clock3 ==
  clock : Inport
  "Reset " : Inport  Port=2
  Memory2 : Memory
  NOT1 : Logic  Operator=NOT  IconShape=distinctive  AllPortsSameDT=off  OutDataTypeStr=boolean
  Product1 : Product
  Triggered Subsystem1 : Subsystem  TreatAsAtomicUnit=on
  T : Outport  VectorParamsAs1DForOutWhenUnconnected=off
  wires:
  Memory2/1 -> Triggered Subsystem1/1(In1)
  Product1/1 -> T/1, Memory2/1
  "Reset "/1 -> NOT1/1
  Triggered Subsystem1/1(Out1) -> Product1/1
  NOT1/1 -> Product1/2
  clock/1 -> Triggered Subsystem1/Trigger

== system pattern3x3_training_2023clock/Synapse27/Subsystem ==
  delta_weight : Inport
  before_weight : Inport  Port=2
  Trigger : TriggerPort  VariantControl=(inherit)  PortDimensions=1
  Sum : Sum  Inputs=|++
  weight : Outport
  wires:
  delta_weight/1 -> Sum/1
  Sum/1 -> weight/1
  before_weight/1 -> Sum/2

== system pattern3x3_training_2023clock/Synapse28/Clock1 ==
  clock : Inport
  "Reset " : Inport  Port=2
  Memory2 : Memory
  NOT1 : Logic  Operator=NOT  IconShape=distinctive  AllPortsSameDT=off  OutDataTypeStr=boolean
  Product1 : Product
  Triggered Subsystem1 : Subsystem  TreatAsAtomicUnit=on
  T : Outport  VectorParamsAs1DForOutWhenUnconnected=off
  wires:
  Memory2/1 -> Triggered Subsystem1/1(In1)
  Product1/1 -> T/1, Memory2/1
  "Reset "/1 -> NOT1/1
  Triggered Subsystem1/1(Out1) -> Product1/1
  NOT1/1 -> Product1/2
  clock/1 -> Triggered Subsystem1/Trigger

== system pattern3x3_training_2023clock/Synapse28/Clock2 ==
  clock : Inport
  "Reset " : Inport  Port=2
  Memory2 : Memory
  NOT1 : Logic  Operator=NOT  IconShape=distinctive  AllPortsSameDT=off  OutDataTypeStr=boolean
  Product1 : Product
  Triggered Subsystem1 : Subsystem  TreatAsAtomicUnit=on
  T : Outport  VectorParamsAs1DForOutWhenUnconnected=off
  wires:
  Memory2/1 -> Triggered Subsystem1/1(In1)
  Product1/1 -> T/1, Memory2/1
  "Reset "/1 -> NOT1/1
  Triggered Subsystem1/1(Out1) -> Product1/1
  NOT1/1 -> Product1/2
  clock/1 -> Triggered Subsystem1/Trigger

== system pattern3x3_training_2023clock/Synapse28/Clock3 ==
  clock : Inport
  "Reset " : Inport  Port=2
  Memory2 : Memory
  NOT1 : Logic  Operator=NOT  IconShape=distinctive  AllPortsSameDT=off  OutDataTypeStr=boolean
  Product1 : Product
  Triggered Subsystem1 : Subsystem  TreatAsAtomicUnit=on
  T : Outport  VectorParamsAs1DForOutWhenUnconnected=off
  wires:
  Memory2/1 -> Triggered Subsystem1/1(In1)
  Product1/1 -> T/1, Memory2/1
  "Reset "/1 -> NOT1/1
  Triggered Subsystem1/1(Out1) -> Product1/1
  NOT1/1 -> Product1/2
  clock/1 -> Triggered Subsystem1/Trigger

== system pattern3x3_training_2023clock/Synapse28/Subsystem ==
  delta_weight : Inport
  before_weight : Inport  Port=2
  Trigger : TriggerPort  VariantControl=(inherit)  PortDimensions=1
  Sum : Sum  Inputs=|++
  weight : Outport
  wires:
  delta_weight/1 -> Sum/1
  Sum/1 -> weight/1
  before_weight/1 -> Sum/2

== system pattern3x3_training_2023clock/Synapse29/Clock1 ==
  clock : Inport
  "Reset " : Inport  Port=2
  Memory2 : Memory
  NOT1 : Logic  Operator=NOT  IconShape=distinctive  AllPortsSameDT=off  OutDataTypeStr=boolean
  Product1 : Product
  Triggered Subsystem1 : Subsystem  TreatAsAtomicUnit=on
  T : Outport  VectorParamsAs1DForOutWhenUnconnected=off
  wires:
  Memory2/1 -> Triggered Subsystem1/1(In1)
  Product1/1 -> T/1, Memory2/1
  "Reset "/1 -> NOT1/1
  Triggered Subsystem1/1(Out1) -> Product1/1
  NOT1/1 -> Product1/2
  clock/1 -> Triggered Subsystem1/Trigger

== system pattern3x3_training_2023clock/Synapse29/Clock2 ==
  clock : Inport
  "Reset " : Inport  Port=2
  Memory2 : Memory
  NOT1 : Logic  Operator=NOT  IconShape=distinctive  AllPortsSameDT=off  OutDataTypeStr=boolean
  Product1 : Product
  Triggered Subsystem1 : Subsystem  TreatAsAtomicUnit=on
  T : Outport  VectorParamsAs1DForOutWhenUnconnected=off
  wires:
  Memory2/1 -> Triggered Subsystem1/1(In1)
  Product1/1 -> T/1, Memory2/1
  "Reset "/1 -> NOT1/1
  Triggered Subsystem1/1(Out1) -> Product1/1
  NOT1/1 -> Product1/2
  clock/1 -> Triggered Subsystem1/Trigger

== system pattern3x3_training_2023clock/Synapse29/Clock3 ==
  clock : Inport
  "Reset " : Inport  Port=2
  Memory2 : Memory
  NOT1 : Logic  Operator=NOT  IconShape=distinctive  AllPortsSameDT=off  OutDataTypeStr=boolean
  Product1 : Product
  Triggered Subsystem1 : Subsystem  TreatAsAtomicUnit=on
  T : Outport  VectorParamsAs1DForOutWhenUnconnected=off
  wires:
  Memory2/1 -> Triggered Subsystem1/1(In1)
  Product1/1 -> T/1, Memory2/1
  "Reset "/1 -> NOT1/1
  Triggered Subsystem1/1(Out1) -> Product1/1
  NOT1/1 -> Product1/2
  clock/1 -> Triggered Subsystem1/Trigger

== system pattern3x3_training_2023clock/Synapse29/Subsystem ==
  delta_weight : Inport
  before_weight : Inport  Port=2
  Trigger : TriggerPort  VariantControl=(inherit)  PortDimensions=1
  Sum : Sum  Inputs=|++
  weight : Outport
  wires:
  delta_weight/1 -> Sum/1
  Sum/1 -> weight/1
  before_weight/1 -> Sum/2

== system pattern3x3_training_2023clock/Synapse3/Clock1 ==
  clock : Inport
  "Reset " : Inport  Port=2
  Memory2 : Memory
  NOT1 : Logic  Operator=NOT  IconShape=distinctive  AllPortsSameDT=off  OutDataTypeStr=boolean
  Product1 : Product
  Triggered Subsystem1 : Subsystem  TreatAsAtomicUnit=on
  T : Outport  VectorParamsAs1DForOutWhenUnconnected=off
  wires:
  Memory2/1 -> Triggered Subsystem1/1(In1)
  Product1/1 -> T/1, Memory2/1
  "Reset "/1 -> NOT1/1
  Triggered Subsystem1/1(Out1) -> Product1/1
  NOT1/1 -> Product1/2
  clock/1 -> Triggered Subsystem1/Trigger

== system pattern3x3_training_2023clock/Synapse3/Clock2 ==
  clock : Inport
  "Reset " : Inport  Port=2
  Memory2 : Memory
  NOT1 : Logic  Operator=NOT  IconShape=distinctive  AllPortsSameDT=off  OutDataTypeStr=boolean
  Product1 : Product
  Triggered Subsystem1 : Subsystem  TreatAsAtomicUnit=on
  T : Outport  VectorParamsAs1DForOutWhenUnconnected=off
  wires:
  Memory2/1 -> Triggered Subsystem1/1(In1)
  Product1/1 -> T/1, Memory2/1
  "Reset "/1 -> NOT1/1
  Triggered Subsystem1/1(Out1) -> Product1/1
  NOT1/1 -> Product1/2
  clock/1 -> Triggered Subsystem1/Trigger

== system pattern3x3_training_2023clock/Synapse3/Clock3 ==
  clock : Inport
  "Reset " : Inport  Port=2
  Memory2 : Memory
  NOT1 : Logic  Operator=NOT  IconShape=distinctive  AllPortsSameDT=off  OutDataTypeStr=boolean
  Product1 : Product
  Triggered Subsystem1 : Subsystem  TreatAsAtomicUnit=on
  T : Outport  VectorParamsAs1DForOutWhenUnconnected=off
  wires:
  Memory2/1 -> Triggered Subsystem1/1(In1)
  Product1/1 -> T/1, Memory2/1
  "Reset "/1 -> NOT1/1
  Triggered Subsystem1/1(Out1) -> Product1/1
  NOT1/1 -> Product1/2
  clock/1 -> Triggered Subsystem1/Trigger

== system pattern3x3_training_2023clock/Synapse3/Subsystem ==
  delta_weight : Inport
  before_weight : Inport  Port=2
  Trigger : TriggerPort  VariantControl=(inherit)  PortDimensions=1
  Sum : Sum  Inputs=|++
  weight : Outport
  wires:
  delta_weight/1 -> Sum/1
  Sum/1 -> weight/1
  before_weight/1 -> Sum/2

== system pattern3x3_training_2023clock/Synapse30/Clock1 ==
  clock : Inport
  "Reset " : Inport  Port=2
  Memory2 : Memory
  NOT1 : Logic  Operator=NOT  IconShape=distinctive  AllPortsSameDT=off  OutDataTypeStr=boolean
  Product1 : Product
  Triggered Subsystem1 : Subsystem  TreatAsAtomicUnit=on
  T : Outport  VectorParamsAs1DForOutWhenUnconnected=off
  wires:
  Memory2/1 -> Triggered Subsystem1/1(In1)
  Product1/1 -> T/1, Memory2/1
  "Reset "/1 -> NOT1/1
  Triggered Subsystem1/1(Out1) -> Product1/1
  NOT1/1 -> Product1/2
  clock/1 -> Triggered Subsystem1/Trigger

== system pattern3x3_training_2023clock/Synapse30/Clock2 ==
  clock : Inport
  "Reset " : Inport  Port=2
  Memory2 : Memory
  NOT1 : Logic  Operator=NOT  IconShape=distinctive  AllPortsSameDT=off  OutDataTypeStr=boolean
  Product1 : Product
  Triggered Subsystem1 : Subsystem  TreatAsAtomicUnit=on
  T : Outport  VectorParamsAs1DForOutWhenUnconnected=off
  wires:
  Memory2/1 -> Triggered Subsystem1/1(In1)
  Product1/1 -> T/1, Memory2/1
  "Reset "/1 -> NOT1/1
  Triggered Subsystem1/1(Out1) -> Product1/1
  NOT1/1 -> Product1/2
  clock/1 -> Triggered Subsystem1/Trigger

== system pattern3x3_training_2023clock/Synapse30/Clock3 ==
  clock : Inport
  "Reset " : Inport  Port=2
  Memory2 : Memory
  NOT1 : Logic  Operator=NOT  IconShape=distinctive  AllPortsSameDT=off  OutDataTypeStr=boolean
  Product1 : Product
  Triggered Subsystem1 : Subsystem  TreatAsAtomicUnit=on
  T : Outport  VectorParamsAs1DForOutWhenUnconnected=off
  wires:
  Memory2/1 -> Triggered Subsystem1/1(In1)
  Product1/1 -> T/1, Memory2/1
  "Reset "/1 -> NOT1/1
  Triggered Subsystem1/1(Out1) -> Product1/1
  NOT1/1 -> Product1/2
  clock/1 -> Triggered Subsystem1/Trigger

== system pattern3x3_training_2023clock/Synapse30/Subsystem ==
  delta_weight : Inport
  before_weight : Inport  Port=2
  Trigger : TriggerPort  VariantControl=(inherit)  PortDimensions=1
  Sum : Sum  Inputs=|++
  weight : Outport
  wires:
  delta_weight/1 -> Sum/1
  Sum/1 -> weight/1
  before_weight/1 -> Sum/2

== system pattern3x3_training_2023clock/Synapse31/Clock1 ==
  clock : Inport
  "Reset " : Inport  Port=2
  Memory2 : Memory
  NOT1 : Logic  Operator=NOT  IconShape=distinctive  AllPortsSameDT=off  OutDataTypeStr=boolean
  Product1 : Product
  Triggered Subsystem1 : Subsystem  TreatAsAtomicUnit=on
  T : Outport  VectorParamsAs1DForOutWhenUnconnected=off
  wires:
  Memory2/1 -> Triggered Subsystem1/1(In1)
  Product1/1 -> T/1, Memory2/1
  "Reset "/1 -> NOT1/1
  Triggered Subsystem1/1(Out1) -> Product1/1
  NOT1/1 -> Product1/2
  clock/1 -> Triggered Subsystem1/Trigger

== system pattern3x3_training_2023clock/Synapse31/Clock2 ==
  clock : Inport
  "Reset " : Inport  Port=2
  Memory2 : Memory
  NOT1 : Logic  Operator=NOT  IconShape=distinctive  AllPortsSameDT=off  OutDataTypeStr=boolean
  Product1 : Product
  Triggered Subsystem1 : Subsystem  TreatAsAtomicUnit=on
  T : Outport  VectorParamsAs1DForOutWhenUnconnected=off
  wires:
  Memory2/1 -> Triggered Subsystem1/1(In1)
  Product1/1 -> T/1, Memory2/1
  "Reset "/1 -> NOT1/1
  Triggered Subsystem1/1(Out1) -> Product1/1
  NOT1/1 -> Product1/2
  clock/1 -> Triggered Subsystem1/Trigger

== system pattern3x3_training_2023clock/Synapse31/Clock3 ==
  clock : Inport
  "Reset " : Inport  Port=2
  Memory2 : Memory
  NOT1 : Logic  Operator=NOT  IconShape=distinctive  AllPortsSameDT=off  OutDataTypeStr=boolean
  Product1 : Product
  Triggered Subsystem1 : Subsystem  TreatAsAtomicUnit=on
  T : Outport  VectorParamsAs1DForOutWhenUnconnected=off
  wires:
  Memory2/1 -> Triggered Subsystem1/1(In1)
  Product1/1 -> T/1, Memory2/1
  "Reset "/1 -> NOT1/1
  Triggered Subsystem1/1(Out1) -> Product1/1
  NOT1/1 -> Product1/2
  clock/1 -> Triggered Subsystem1/Trigger

== system pattern3x3_training_2023clock/Synapse31/Subsystem ==
  delta_weight : Inport
  before_weight : Inport  Port=2
  Trigger : TriggerPort  VariantControl=(inherit)  PortDimensions=1
  Sum : Sum  Inputs=|++
  weight : Outport
  wires:
  delta_weight/1 -> Sum/1
  Sum/1 -> weight/1
  before_weight/1 -> Sum/2

== system pattern3x3_training_2023clock/Synapse32/Clock1 ==
  clock : Inport
  "Reset " : Inport  Port=2
  Memory2 : Memory
  NOT1 : Logic  Operator=NOT  IconShape=distinctive  AllPortsSameDT=off  OutDataTypeStr=boolean
  Product1 : Product
  Triggered Subsystem1 : Subsystem  TreatAsAtomicUnit=on
  T : Outport  VectorParamsAs1DForOutWhenUnconnected=off
  wires:
  Memory2/1 -> Triggered Subsystem1/1(In1)
  Product1/1 -> T/1, Memory2/1
  "Reset "/1 -> NOT1/1
  Triggered Subsystem1/1(Out1) -> Product1/1
  NOT1/1 -> Product1/2
  clock/1 -> Triggered Subsystem1/Trigger

== system pattern3x3_training_2023clock/Synapse32/Clock2 ==
  clock : Inport
  "Reset " : Inport  Port=2
  Memory2 : Memory
  NOT1 : Logic  Operator=NOT  IconShape=distinctive  AllPortsSameDT=off  OutDataTypeStr=boolean
  Product1 : Product
  Triggered Subsystem1 : Subsystem  TreatAsAtomicUnit=on
  T : Outport  VectorParamsAs1DForOutWhenUnconnected=off
  wires:
  Memory2/1 -> Triggered Subsystem1/1(In1)
  Product1/1 -> T/1, Memory2/1
  "Reset "/1 -> NOT1/1
  Triggered Subsystem1/1(Out1) -> Product1/1
  NOT1/1 -> Product1/2
  clock/1 -> Triggered Subsystem1/Trigger

== system pattern3x3_training_2023clock/Synapse32/Clock3 ==
  clock : Inport
  "Reset " : Inport  Port=2
  Memory2 : Memory
  NOT1 : Logic  Operator=NOT  IconShape=distinctive  AllPortsSameDT=off  OutDataTypeStr=boolean
  Product1 : Product
  Triggered Subsystem1 : Subsystem  TreatAsAtomicUnit=on
  T : Outport  VectorParamsAs1DForOutWhenUnconnected=off
  wires:
  Memory2/1 -> Triggered Subsystem1/1(In1)
  Product1/1 -> T/1, Memory2/1
  "Reset "/1 -> NOT1/1
  Triggered Subsystem1/1(Out1) -> Product1/1
  NOT1/1 -> Product1/2
  clock/1 -> Triggered Subsystem1/Trigger

== system pattern3x3_training_2023clock/Synapse32/Subsystem ==
  delta_weight : Inport
  before_weight : Inport  Port=2
  Trigger : TriggerPort  VariantControl=(inherit)  PortDimensions=1
  Sum : Sum  Inputs=|++
  weight : Outport
  wires:
  delta_weight/1 -> Sum/1
  Sum/1 -> weight/1
  before_weight/1 -> Sum/2

== system pattern3x3_training_2023clock/Synapse33/Clock1 ==
  clock : Inport
  "Reset " : Inport  Port=2
  Memory2 : Memory
  NOT1 : Logic  Operator=NOT  IconShape=distinctive  AllPortsSameDT=off  OutDataTypeStr=boolean
  Product1 : Product
  Triggered Subsystem1 : Subsystem  TreatAsAtomicUnit=on
  T : Outport  VectorParamsAs1DForOutWhenUnconnected=off
  wires:
  Memory2/1 -> Triggered Subsystem1/1(In1)
  Product1/1 -> T/1, Memory2/1
  "Reset "/1 -> NOT1/1
  Triggered Subsystem1/1(Out1) -> Product1/1
  NOT1/1 -> Product1/2
  clock/1 -> Triggered Subsystem1/Trigger

== system pattern3x3_training_2023clock/Synapse33/Clock2 ==
  clock : Inport
  "Reset " : Inport  Port=2
  Memory2 : Memory
  NOT1 : Logic  Operator=NOT  IconShape=distinctive  AllPortsSameDT=off  OutDataTypeStr=boolean
  Product1 : Product
  Triggered Subsystem1 : Subsystem  TreatAsAtomicUnit=on
  T : Outport  VectorParamsAs1DForOutWhenUnconnected=off
  wires:
  Memory2/1 -> Triggered Subsystem1/1(In1)
  Product1/1 -> T/1, Memory2/1
  "Reset "/1 -> NOT1/1
  Triggered Subsystem1/1(Out1) -> Product1/1
  NOT1/1 -> Product1/2
  clock/1 -> Triggered Subsystem1/Trigger
